simulink model "Observer"  (Simulink 8.3)
settings: Solver=FixedStepDiscrete  SolverMode=SingleTasking  StartTime=0.0  StopTime=positions.time(end)  FixedStep=Ts  RelTol=1e-3
PreLoadFcn:
  | Ts=1e-2;
libraries: dspbuff3 x1, dspsrcs4 x1
settings Model: Creator=Carchesion  LastModifiedBy=makaveli
settings DataIOCC: LimitDataPoints=off  SaveOutput=off  SignalLogging=off  SaveTime=off
settings OptimizationCC: ExpressionDepthLimit=2147483647  InitFltsAndDblsToZero=on
settings DebuggingCC: FcnCallInpInsideContextMsg=UseLocalSettings
settings SFSimCC: SimParseCustomCode=off

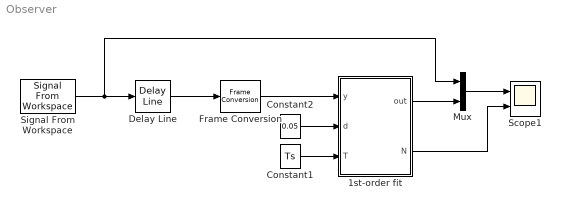
== system Observer ==
  1st-order fit : MATLAB Function  TreatAsAtomicUnit=on
  Constant1 : Constant  Value=Ts
  Constant2 : Constant  Value=0.05
  Delay Line : dspbuff3/Delay Line  siz=64  ic=0  directfeed=off  enable_output=off  hold_output=off  TreatMby1Signals=M channels (this choice will be removed - see release notes)
  Frame Conversion : FrameConversion  OutFrame=Sample-based
  Mux : Mux  Inputs=2
  Scope1 : Scope  NumInputPorts=2
      settings: TimeRange=53.45  YMin=-1~0  YMax=1~65
  Signal From Workspace : dspsrcs4/Signal From Workspace  X=posInRad  Ts=Ts  nsamps=1  OutputAfterFinalValue=Setting to zero  ignoreOrWarnInputAndFrameLengths=off
  wires:
  Delay Line/1 -> Frame Conversion/1
  Constant1/1 -> 1st-order fit/3(T)
  Constant2/1 -> 1st-order fit/2(d)
  Frame Conversion/1 -> 1st-order fit/1(y)
  Mux/1 -> Scope1/1
  1st-order fit/2(N) -> Scope1/2
  1st-order fit/1(out) -> Mux/2
  Signal From Workspace/1 -> Mux/1, Delay Line/1

== matlab function 1st-order fit ==
  data: y input double; out output double; d input double; T input double; N output double
function [out,N]=fcn(y,d,T)
%#ok<*NASGU>

coder.extrinsic('polyfitHelper');

persistent n;
if isempty(n)
    n=1;
end

L=length(y);
pos=zeros(1,2);
Ly=0;
N=n;

for j=max(1,n-1):min(n+1,L-1)
    pos=polyfitHelper(y,1,T,j);

    finish=false;
    for i=0:j
        Ly=polyval(pos,i*T);
        if abs(y(L-j+i)-Ly)>d
            finish=true;
            break;
        end
    end
    
    if finish
        N=j;
        break;
    end
    N=j;
end

out=pos(1);
n=N;
